simulink model "slink5"  (R2024a)
settings: Solver=FixedStepAuto  StartTime=0.0  StopTime=inf  RelTol=1e-3
libraries: instrumentseriallib x2
settings Model: Creator=alexe  LastModifiedBy=alexe

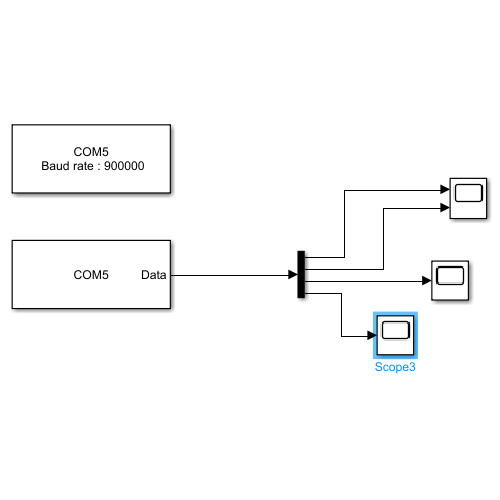
[thumbnail: Simulink's stored preview of the top-level diagram]
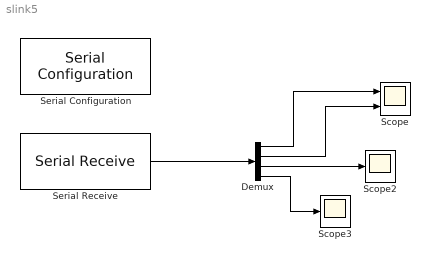
== system slink5 ==
  Demux : Demux
  Scope : Scope  NumInputPorts=2
  Scope2 : Scope
  Scope3 : Scope
  Serial Configuration : instrumentseriallib/Serial Configuration  Priority=-200000  PortSel=COM5  Port=COM5  ComPort=COM5  BaudRate=900000  DataBits=8  Parity=none  StopBits=1  ByteOrder=little-endian  FlowControl=none  Timeout=10  SimulateUsing=Interpreted execution  BlockInModel=on  aMode=1
      settings: LibrarySourceBlock=c2000lib/Host Communication/Serial Configuration
  Serial Receive : instrumentseriallib/Serial Receive  Priority=1  PortSel=COM5  Port=COM5  ComPort=COM5  DataType=int16  SaveDataType=uint8  ToggleHeader=on  Header=[170 170]  ToggleDataSize=on  DataSize=[4 1]  ToggleTerminator=on  Terminator=Custom terminator  CustomTerminator=[187 187]  InputFormat=Column major  EnableBlockingMode=on  ActionDataUnavailable=Error  ActionWhenDataUnavailable=Error  CustomValue=0  SampleTime=0.001  SimulateUsing=Interpreted execution  BlockInModel=on  aMode=1
      settings: LibrarySourceBlock=c2000lib/Host Communication/Serial Receive
  wires:
  Serial Receive/1 -> Demux/1
  Demux/1 -> Scope/1
  Demux/2 -> Scope/2
  Demux/3 -> Scope2/1
  Demux/4 -> Scope3/1
